simulink model "Vorlage"  (R2024a)
settings: Solver=ode45  StartTime=0.0  StopTime=1  FixedStep=1e-2  RelTol=1e-4  AbsTol=1e-4
values from neighbouring files (symbols this model uses):
  Kp = 9.8    [ITAE_Plots_PT2_limitations Rechenbeispiel.m]
  Td = 0.01    [ITAE_Plots_PT2_limitations Rechenbeispiel.m]
  Ti = 0.11    [ITAE_Plots_PT2_limitations Rechenbeispiel.m]
libraries: cstblocks x1
settings Model: Creator=bhir  LastModifiedBy=Flo
settings SolverCC: AlgebraicLoopSolver=TrustRegion
settings DataIOCC: ReturnWorkspaceOutputs=off
settings DebuggingCC: UnconnectedInputMsg=warning  UnconnectedOutputMsg=warning  UnconnectedLineMsg=warning  ArithmeticOperatorsInVariantConditions=warning
settings SFSimCC: SimUseLocalCustomCode=off  CustomCodeUndefinedFunction=UseInterfaceOnly
settings RTWCC: RTWUseLocalCustomCode=off  GPUComputeCapability=3.5  DLArmComputeVersion=19.05
settings CodeAppCC: StateflowObjectComments=on

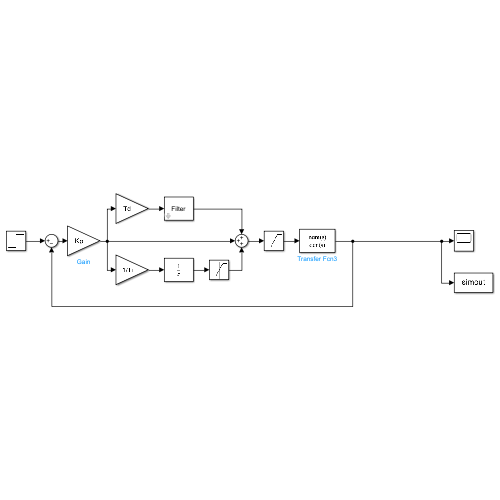
[thumbnail: Simulink's stored preview of the top-level diagram]
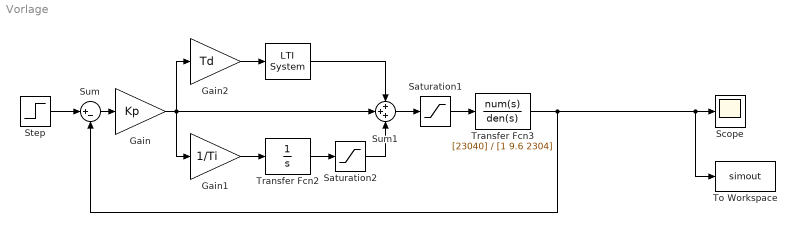
== system Vorlage ==
  " " : cstblocks/LTI System  sys=Filter  IC=[]  PadeOrder=0
  Gain : Gain  Gain=Kp
  Gain1 : Gain  Gain=1/Ti
  Gain2 : Gain  Gain=Td
  Saturation1 : Saturate  UpperLimit=4  LowerLimit=-4
  Saturation2 : Saturate  UpperLimit=4  LowerLimit=-4
  Scope : Scope
  Step : Step  Time=0  SampleTime=0
  Sum : Sum  Inputs=|+-
  Sum1 : Sum  Inputs=+++
  To Workspace : ToWorkspace  VariableName=simout  SaveFormat=Structure With Time  SampleTime=-1
  Transfer Fcn2 : TransferFcn  Denominator=[1 0]
  Transfer Fcn3 : TransferFcn  Numerator=[23040]  Denominator=[1 9.6 2304]
  wires:
  Step/1 -> Sum/1
  Sum/1 -> Gain/1
  Gain1/1 -> Transfer Fcn2/1
  Gain/1 -> Gain2/1, Sum1/2, Gain1/1
  " "/1 -> Sum1/1
  Gain2/1 -> " "/1
  Transfer Fcn3/1 -> To Workspace/1, Scope/1, Sum/2
  Sum1/1 -> Saturation1/1
  Transfer Fcn2/1 -> Saturation2/1
  Saturation2/1 -> Sum1/3
  Saturation1/1 -> Transfer Fcn3/1
